simulink model "mpcLKAsystem_EvolvingPath"  (R2022a)
settings: Solver=VariableStepAuto  StartTime=0.0  StopTime=15  RelTol=1e-3
values from neighbouring files (symbols this model uses):
  Cf = 19000    [Workspace.mat]
  chg = [0.001 0.002 0.003 0.004 0.005 0.006 0.007 0.008 0.009 0.01 0.011 0.012 ... (40 elements, 1x40)]    [chang.mat]
  Cr = 33000    [Workspace.mat]
  Iz = 2875    [Workspace.mat]
  lf = 1.2    [Workspace.mat]
  lr = 1.6    [Workspace.mat]
  m = 1575    [Workspace.mat]
  Ts = 0.1    [Workspace.mat]
  Vx = 15    [Workspace.mat]
libraries: mpcadaslib x1
settings Model: Creator=The MathWorks, Inc.  LastModifiedBy=Omkar
settings SolverCC: AlgebraicLoopSolver=TrustRegion
settings DataIOCC: ReturnWorkspaceOutputs=off
settings DebuggingCC: UnconnectedInputMsg=warning  UnconnectedOutputMsg=warning  UnconnectedLineMsg=warning  SFMachineParentedDataDiag=warning  ArithmeticOperatorsInVariantConditions=warning
settings SFSimCC: SimUseLocalCustomCode=off  CustomCodeUndefinedFunction=UseInterfaceOnly
settings RTWCC: RTWUseLocalCustomCode=off
settings CodeAppCC: StateflowObjectComments=on
settings SimscapeCC: SimscapeNormalizeSystem=off

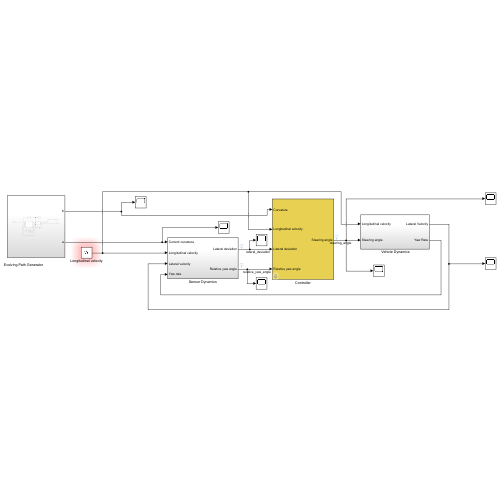
[thumbnail: Simulink's stored preview of the top-level diagram]
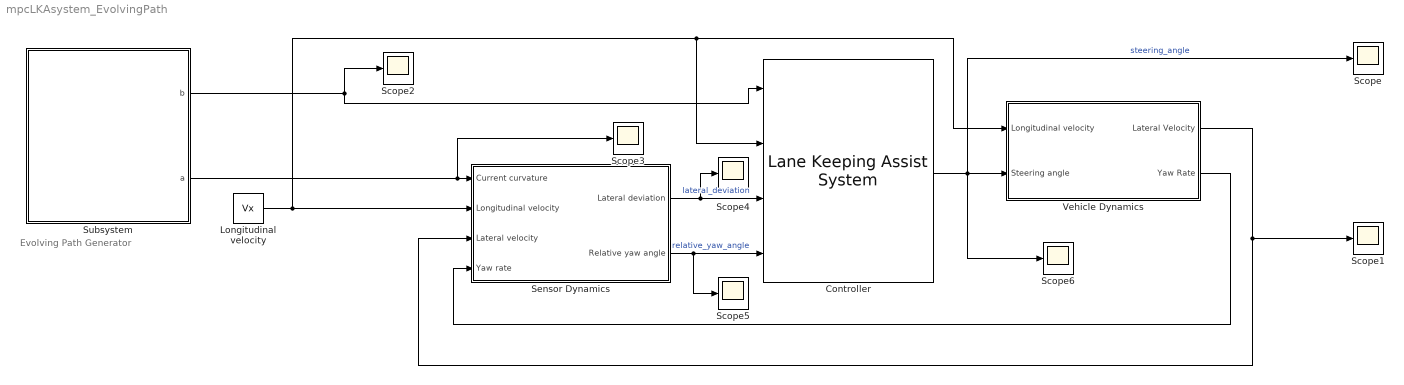
== system mpcLKAsystem_EvolvingPath ==
  note: Evolving Path Generator
  " Vehicle Dynamics" : Subsystem
  Controller : mpcadaslib/Lane Keeping Assist System  ModelType=Use vehicle parameters  VehicleMass=1575  VehicleYawInertia=2875  LengthToFront=1.2  LengthToRear=1.6  FrontTireStiffness=19000  RearTireStiffness=33000  EgoModelMatrixA=[-4.4021 ,-12.4603;1.3913,-5.1868]  EgoModelMatrixB=[24.1270;15.8609]  EgoModelMatrixC=[1,0;0,1]  InitialLongVel=15  TransportLag=0  MinSteering=-0.26  umin_ext=off  MaxSteering=0.26  umax_ext=off  Ts=0.1  PredictionHorizon=10  ControllerBehavior=0.5  suboptimal=off  maxiter=10  datatypeopt=double  optmode=off  trackmode=off
      settings: SourceProductBaseCode=MP
  Longitudinal velocity : Constant  Value=Vx  SampleTime=Ts
  Scope{,1..6} (7 alike) : Scope
  Sensor Dynamics : Subsystem
  Subsystem : Subsystem
  wires:
  " Vehicle Dynamics"/2(Yaw Rate) -> Sensor Dynamics/4(Yaw rate)
  " Vehicle Dynamics"/1(Lateral Velocity) -> Sensor Dynamics/3(Lateral velocity), Scope1/1
  Sensor Dynamics/1(Lateral deviation) -> Scope4/1, Controller/3  "lateral_deviation"
  Sensor Dynamics/2(Relative yaw angle) -> Scope5/1, Controller/4  "relative_yaw_angle"
  Longitudinal velocity/1 -> Controller/2, " Vehicle Dynamics"/1(Longitudinal velocity), Sensor Dynamics/2(Longitudinal velocity)
  Controller/1 -> Scope6/1, Scope/1, " Vehicle Dynamics"/2(Steering angle)  "steering_angle"
  Subsystem/2(a) -> Scope3/1, Sensor Dynamics/1(Current curvature)
  Subsystem/1(b) -> Controller/1, Scope2/1

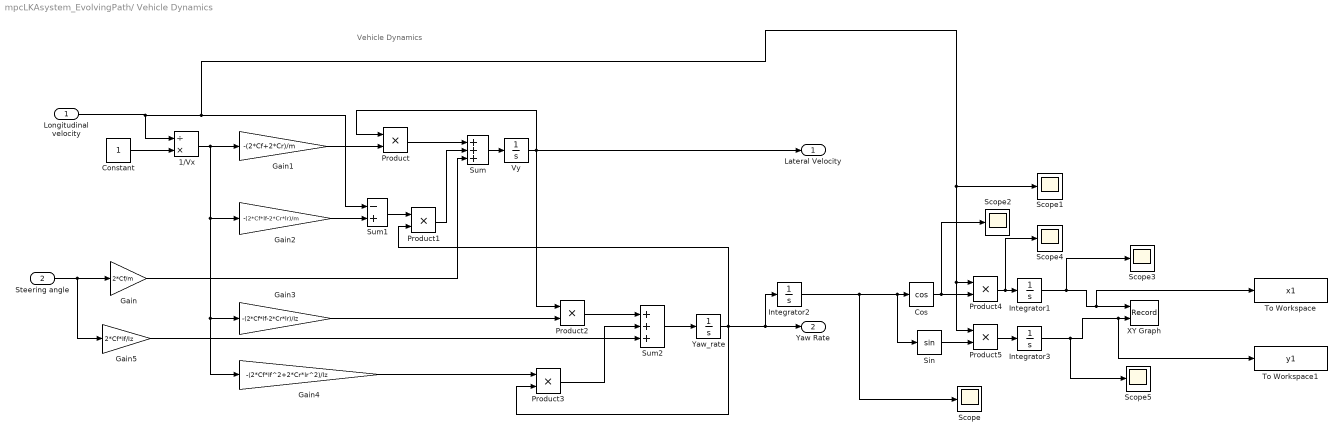
== system mpcLKAsystem_EvolvingPath/ Vehicle Dynamics ==
  note: Vehicle Dynamics
  Longitudinal velocity : Inport
  Steering angle : Inport  Port=2
  1/Vx : Product  Inputs=/*
  Constant : Constant
  Cos : Trigonometry  Operator=cos
  Gain : Gain  Gain=2*Cf/m
  Gain1 : Gain  Gain=-(2*Cf+2*Cr)/m
  Gain2 : Gain  Gain=-(2*Cf*lf-2*Cr*lr)/m
  Gain3 : Gain  Gain=-(2*Cf*lf-2*Cr*lr)/Iz
  Gain4 : Gain  Gain=-(2*Cf*lf^2+2*Cr*lr^2)/Iz
  Gain5 : Gain  Gain=2*Cf*lf/Iz
  Integrator1 : Integrator
  Integrator2 : Integrator
  Integrator3 : Integrator
  Product{,1..5} (6 alike) : Product
  Scope{,1..5} (6 alike) : Scope
  Sin : Trigonometry
  Sum : Sum  Inputs=+++
  Sum1 : Sum  Inputs=-+
  Sum2 : Sum  Inputs=+++
  To Workspace : ToWorkspace  VariableName=x1  SampleTime=0.1
  To Workspace1 : ToWorkspace  VariableName=y1  SampleTime=0.1
  Vy : Integrator
  XY Graph : Record  FileSettingsInternal="{\"entries\":[{\"content\":{\"excelSettings\":{\"content\":{},\"type\":\"Streamout.ExcelSettings\"}},\"type\":\"Streamout.FileSettingStorage\",\"uuid\":\"51cf17a2-4609-48d9-b522-40c7f1266197\"}],\"packageUris\":[\"http://schema.mathworks.com/mf0/streamout_blocks/R2020a\"],\"version\":\"1.0\"}"  Layout=[1 1]  SignalsInternal="{\"entries\":[{\"content\":{\"signals\":[{\"content\":{\"blockPath\":[\"mpcLKAsystem_EvolvingPath/ Vehicle Dynamics/XY Graph\"],\"channel\":[],\"dimensions\":[1],\"domain\":\"mpcLKAsystem_EvolvingPath/ Vehicle Dynamics/XY Graph\",\"lineColor\":\"#a2142f\",\"plots\":[1],\"port\":1,\"sid\":[\"\"],\"signalID\":283,\"signalName\":\"Integrator1\"},\"type\":\"RecordBlkView.Signal\",\"uuid\":\"312384ec-e516-499c-bf7b-178629121b22\"},{\"content\":{\"blockPath\":[\"mpcLKAsystem_EvolvingPath/ Vehicle Dynamics/XY Graph\"],\"channel\":[],\"dimensions\":[1],\"domain\":\"mpcLKAsystem_EvolvingPath/ Vehicle Dynamics/XY Graph\",\"lineColor\":\"#139fff\",\"plots\":[1],\"port\":2,\"sid\":[\"\"],\"signalID\":287,\"signalName\":\"Integrator3\"},\"type\":\"RecordBlkView.Signal\",\"uuid\":\"4a10691f-ad62-4491-91cc-c4262014cd1f\"}]},\"type\":\"RecordBlkView.InputSignals\",\"uuid\":\"d44e5f54-55db-4b5c-90ef-f1a02158aa35\"}],\"packageUris\":[\"http://schema.mathworks.com/mf0/streamout_blocks/R2020a\"],\"version\":\"1.0\"}"  VisualizationBindings="{\"xyplotplugin\":{\"info\":[{\"series\":[{\"bindingParametersList\":[{\"parameter\":\"X-Axis\",\"signalID\":283,\"signalName\":\"Integrator1\"},{\"parameter\":\"Y-Axis\",\"signalID\":287,\"signalName\":\"Integrator3\"}],\"seriesID\":48544}],\"subplotID\":1}]}}"  CompatibilityTag=XY
  "Yaw_rate " : Integrator
  Lateral Velocity : Outport  VectorParamsAs1DForOutWhenUnconnected=off
  Yaw Rate : Outport  Port=2  VectorParamsAs1DForOutWhenUnconnected=off
  wires:
  Sum2/1 -> "Yaw_rate "/1
  Gain2/1 -> Sum1/2
  Gain4/1 -> Product3/1
  Constant/1 -> 1/Vx/2
  Gain3/1 -> Product2/2
  1/Vx/1 -> Gain4/1, Gain3/1, Gain2/1, Gain1/1
  Product2/1 -> Sum2/1
  Product3/1 -> Sum2/2
  Gain5/1 -> Sum2/3
  Sum1/1 -> Product1/1
  "Yaw_rate "/1 -> Product3/2, Integrator2/1, Yaw Rate/1, Product1/2
  Gain/1 -> Sum/3
  Steering angle/1 -> Gain/1, Gain5/1
  Gain1/1 -> Product/2
  Product/1 -> Sum/1
  Vy/1 -> Product/1, Lateral Velocity/1, Product2/1
  Sum/1 -> Vy/1
  Longitudinal velocity/1 -> Scope1/1, Product5/1, Product4/1, Sum1/1, 1/Vx/1
  Product1/1 -> Sum/2
  Integrator2/1 -> Scope/1, Sin/1, Cos/1
  Cos/1 -> Scope2/1, Product4/2
  Product4/1 -> Scope4/1, Integrator1/1
  Sin/1 -> Product5/2
  Product5/1 -> Integrator3/1
  Integrator3/1 -> Scope5/1, To Workspace1/1, XY Graph/2
  Integrator1/1 -> Scope3/1, To Workspace/1, XY Graph/1

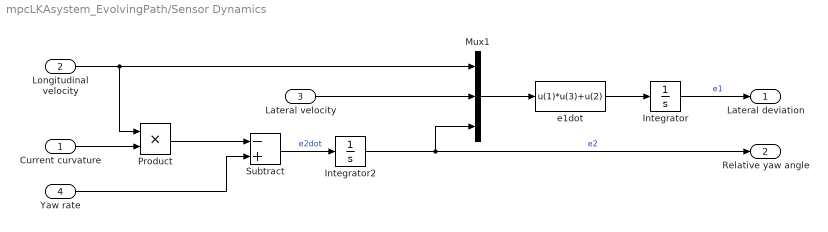
== system mpcLKAsystem_EvolvingPath/Sensor Dynamics ==
  Current curvature : Inport
  Longitudinal velocity : Inport  Port=2
  Lateral velocity : Inport  Port=3
  Yaw rate : Inport  Port=4
  Integrator : Integrator
  Integrator2 : Integrator
  Mux1 : Mux  Inputs=[1 1 1]
  Product : Product
  Subtract : Sum  Inputs=-+
  e1dot : Fcn  Expr=u(1)*u(3)+u(2)
  Lateral deviation : Outport  VectorParamsAs1DForOutWhenUnconnected=off
  Relative yaw angle : Outport  Port=2  VectorParamsAs1DForOutWhenUnconnected=off
  wires:
  Current curvature/1 -> Product/2
  Integrator2/1 -> Mux1/3, Relative yaw angle/1  "e2"
  Mux1/1 -> e1dot/1
  e1dot/1 -> Integrator/1
  Longitudinal velocity/1 -> Product/1, Mux1/1
  Lateral velocity/1 -> Mux1/2
  Integrator/1 -> Lateral deviation/1  "e1"
  Product/1 -> Subtract/1
  Yaw rate/1 -> Subtract/2
  Subtract/1 -> Integrator2/1  "e2dot"

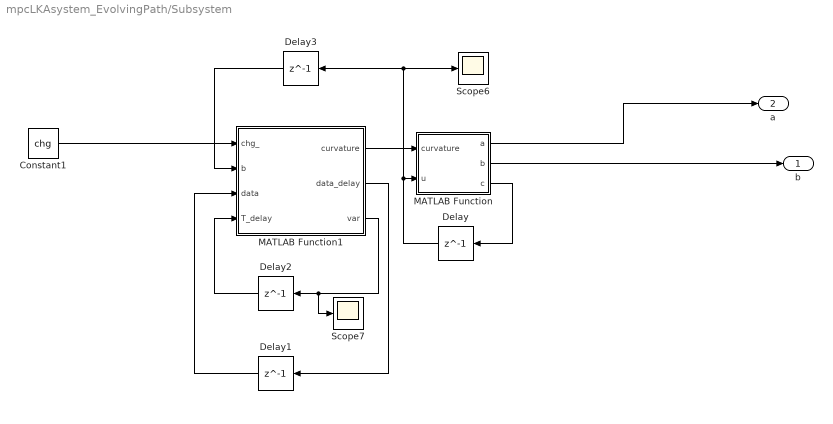
== system mpcLKAsystem_EvolvingPath/Subsystem ==
  Constant1 : Constant  Value=chg  VectorParams1D=off
  Delay : Delay  DelayLength=1  InitialCondition=1
  Delay1 : Delay  DelayLength=1
  Delay2 : Delay  DelayLength=1
  Delay3 : Delay  DelayLength=1
  MATLAB Function : MATLAB Function  TreatAsAtomicUnit=on
  MATLAB Function1 : MATLAB Function  TreatAsAtomicUnit=on
  Scope6 : Scope
  Scope7 : Scope
  b : Outport
  a : Outport  Port=2
  wires:
  Delay/1 -> Scope6/1, Delay3/1, MATLAB Function/2(u)
  MATLAB Function1/2(data_delay) -> Delay1/1
  MATLAB Function1/3(var) -> Scope7/1, Delay2/1
  MATLAB Function1/1(curvature) -> MATLAB Function/1(curvature)
  MATLAB Function/3(c) -> Delay/1
  Delay2/1 -> MATLAB Function1/4(T_delay)
  Delay3/1 -> MATLAB Function1/2(b)
  Constant1/1 -> MATLAB Function1/1(chg_)
  Delay1/1 -> MATLAB Function1/3(data)
  MATLAB Function/2(b) -> b/1
  MATLAB Function/1(a) -> a/1

== matlab function mpcLKAsystem_EvolvingPath/Subsystem/MATLAB Function1 ==
  settings: updateMethod=DISCRETE
  data: chg_ input; b input; curvature output; data_delay output; data input; T_delay input; var output
function [curvature,data_delay,var] = fcn(chg_, b, data,T_delay)
curvature=zeros(1,151);
Ncurv=curvature;
data_delay=data;
var=T_delay;
if data_delay==0

    var = randi([21, 50], 1)
    %randi([21, 40], 1)
    %bkhb=randi([21, 90], 1)
    data_delay=1+data;
end
if data_delay==1
    Ncurv(var:(var+39))=chg_
end

if (b+12)>=var
    curvature=Ncurv;
end

end

== matlab function mpcLKAsystem_EvolvingPath/Subsystem/MATLAB Function ==
  data: curvature input; a output; b output; c output; u input
function [a, b, c] = fcn(curvature, u)
c=u;
d=u;
g=curvature;
a=g(c);
b=zeros(1,11);
for i=1:11
    if d<152
        b(i)=g(d);
    else
        b(i)=g(151)
    end
    d=1+d;
end

c=1+c;
end
